simulink model "Toggle_On_RisingEdge_Fixed"  (R2025a)
settings: Solver=VariableStepAuto  StartTime=0.0  StopTime=10.0  RelTol=1e-3
settings Model: Creator=mahij  LastModifiedBy=mahij

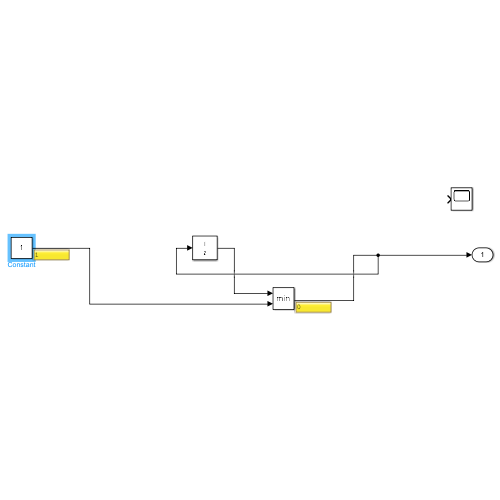
[thumbnail: Simulink's stored preview of the top-level diagram]
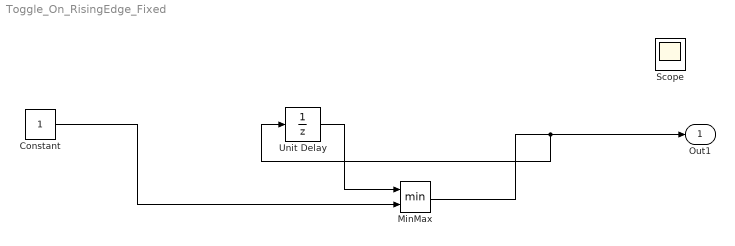
== system Toggle_On_RisingEdge_Fixed ==
  Constant : Constant
  MinMax : MinMax  Inputs=2
  Scope : Scope
      settings: ActiveDisplayYMinimum=-1  ActiveDisplayYMaximum=1
  Unit Delay : UnitDelay  SampleTime=-1  HasFrameUpgradeWarning=on
  Out1 : Outport
  wires:
  Constant/1 -> MinMax/2
  Unit Delay/1 -> MinMax/1
  MinMax/1 -> Unit Delay/1, Out1/1
